simulink model "comp_offset_input_cancel"  (R2018b)
settings: Solver=VariableStepAuto  StartTime=0.0  StopTime=10.0  RelTol=1e-3
libraries: simulink x1
settings Model: Creator=iamcy  LastModifiedBy=iamcy

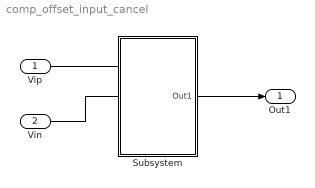
== system comp_offset_input_cancel ==
  Vip : Inport
  Vin : Inport  Port=2
  Subsystem : Subsystem
  Out1 : Outport
  wires:
  Vip/1 -> ?
  Vin/1 -> ?
  Subsystem/1(Out1) -> Out1/1

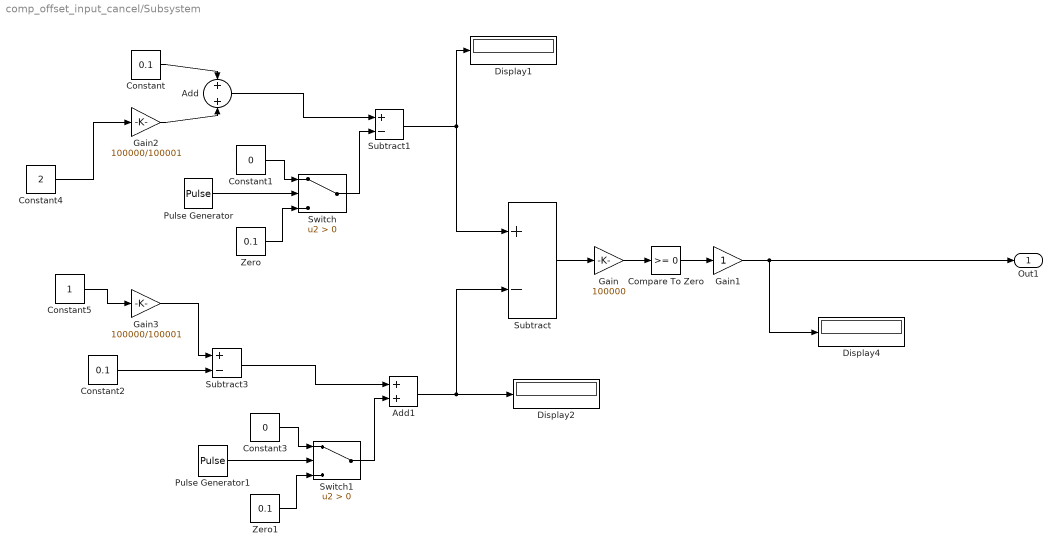
== system comp_offset_input_cancel/Subsystem ==
  Add : Sum  Inputs=2
  Add1 : Sum
  Compare To Zero : simulink/Logic and Bit Operations/Compare To Zero  relop=>=  OutDataTypeStr=boolean
  Constant : Constant  Value=0.1
  Constant1 : Constant  Value=0
  Constant2 : Constant  Value=0.1
  Constant3 : Constant  Value=0
  Constant4 : Constant  Value=2
  Constant5 : Constant
  Display1 : Display
  Display2 : Display
  Display4 : Display
  Gain : Gain  Gain=100000
  Gain1 : Gain
  Gain2 : Gain  Gain=100000/100001
  Gain3 : Gain  Gain=100000/100001
  Pulse Generator : DiscretePulseGenerator  PulseType=Time based  Period=10  PulseWidth=5
  Pulse Generator1 : DiscretePulseGenerator  PulseType=Time based  Period=10  PulseWidth=5
  Subtract : Sum  Inputs=+-
  Subtract1 : Sum  Inputs=+-
  Subtract3 : Sum  Inputs=+-
  Switch : Switch  Criteria=u2 > Threshold
  Switch1 : Switch  Criteria=u2 > Threshold
  Zero : Constant  Value=0.1  OutDataTypeStr=Inherit: Inherit via back propagation
  Zero1 : Constant  Value=0.1  OutDataTypeStr=Inherit: Inherit via back propagation
  Out1 : Outport
  wires:
  Compare To Zero/1 -> Gain1/1
  Subtract/1 -> Gain/1
  Gain3/1 -> Subtract3/1
  Add/1 -> Subtract1/1
  Subtract1/1 -> Display1/1, Subtract/1
  Constant2/1 -> Subtract3/2
  Zero1/1 -> Switch1/3
  Switch/1 -> Subtract1/2
  Gain1/1 -> Out1/1, Display4/1
  Add1/1 -> Display2/1, Subtract/2
  Subtract3/1 -> Add1/1
  Gain/1 -> Compare To Zero/1
  Switch1/1 -> Add1/2
  Zero/1 -> Switch/3
  Pulse Generator1/1 -> Switch1/2
  Constant/1 -> Add/1
  Gain2/1 -> Add/2
  Pulse Generator/1 -> Switch/2
  Constant1/1 -> Switch/1
  Constant3/1 -> Switch1/1
  Constant4/1 -> Gain2/1
  Constant5/1 -> Gain3/1
